simulink model "UseBus"  (R2020b)
settings: Solver=VariableStepAuto  StartTime=0.0  StopTime=10.0  RelTol=1e-3
settings Model: Creator=kaebi  LastModifiedBy=kaebi

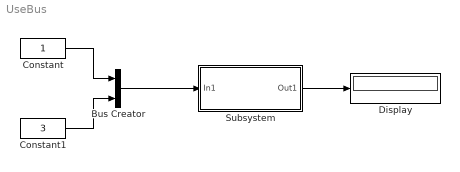
== system UseBus ==
  Bus Creator : BusCreator  Inputs=2
  Constant : Constant
  Constant1 : Constant  Value=3
  Display : Display
  Subsystem : Subsystem
  wires:
  Constant1/1 -> Bus Creator/2
  Constant/1 -> Bus Creator/1
  Bus Creator/1 -> Subsystem/1(In1)
  Subsystem/1(Out1) -> Display/1

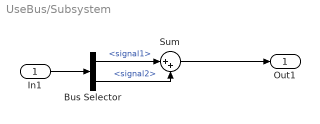
== system UseBus/Subsystem ==
  In1 : Inport  OutDataTypeStr=Bus: InputBus
  Bus Selector : BusSelector  OutputSignals=signal1,signal2
  Sum : Sum  Inputs=|++
  Out1 : Outport
  wires:
  Bus Selector/1 -> Sum/1  "<signal1>"
  Bus Selector/2 -> Sum/2  "<signal2>"
  Sum/1 -> Out1/1
  In1/1 -> Bus Selector/1
